simulink model "Elevator_Group_Final"  (R2020b)
settings: Solver=VariableStepAuto  StartTime=0.0  StopTime=100  RelTol=1e-3
libraries: vrlib x6
settings Model: SimulationMode=accelerator  EnablePacing=on  Creator=eric  LastModifiedBy=eric

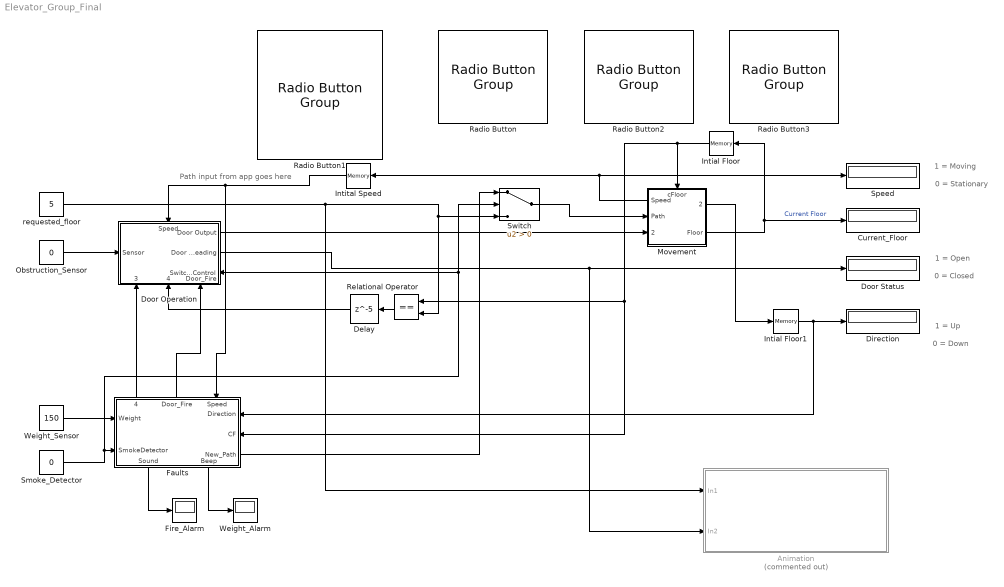
== system Elevator_Group_Final ==
  note: 0 = Closed
  note: 1 = Open
  note: 0 = Stationary
  note: 1 = Moving
  note: 0 = Down
  note: 1 = Up
  note: Path input from app goes here
  Animation : Subsystem  Commented=on
  Current_Floor : Display
  Delay : Delay  DelayLength=5  DelayLengthUpperLimit=1  InitialCondition=5
  Direction : Display
  Door Operation : Subsystem
      settings: PortSchema="{\"entries\":[{\"content\":{\"sides\":[{\"content\":{\"connectorIds\":[\"In1\"]},\"type\":\"ConnectorPlacement.EquallySpacedRectSide\",\"uuid\":\"30977b0a-2af7-4c61-bebb-4ec80410b903\"},{\"content\":{\"connectorIds\":[\"Out1\",\"Out2\",\"In6\"],\"side\":\"RIGHT\"},\"type\":\"ConnectorPlacement.EquallySpacedRectSide\",\"uuid\":\"323388e5-4c35-430e-8d9e-2a05895b747e\"},{\"content\":{\"connectorIds\":[\"In2\"],\"side\":\"TOP\"},\"type\":\"ConnectorPlacement.EquallySpacedRectSide\",\"uuid\":\"9d5d1b04-f04c-4d1c-b5e3-f520ce15ffef\"},{\"content\":{\"connectorIds\":[\"In3\",\"In4\",\"In5\"],\"side\":\"BOTTOM\"},\"type\":\"ConnectorPlacement.EquallySpacedRectSide\",\"uuid\":\"a2796d79-cbcd-43fd-84cb-bc57d429544b\"},{\"content\":{\"connectorIds\":[],\"side\":\"HIDDEN\"},\"type\":\"ConnectorPlacement.EquallySpacedRectSide\",\"uuid\":\"d7ca2218-6b24-4bda-a0e6-55c9b81b1772\"}]},\"type\":\"ConnectorPlacement.EquallySpacedConnector\",\"uuid\":\"8cf9c2d5-6e60-4b33-b84b-36b0ae7fd4c7\"}],\"packageUris\":[\"http://schema.mathworks.com/mf0/Connector/R2020b\"],\"version\":\"1.0\"}"
  Door Status : Display
      settings: Format=decimal (Stored Integer)
  Faults : Subsystem
      settings: PortSchema="{\"entries\":[{\"content\":{\"sides\":[{\"content\":{\"connectorIds\":[\"In1\",\"In2\"]},\"type\":\"ConnectorPlacement.EquallySpacedRectSide\",\"uuid\":\"b542c6e3-be07-4424-9acd-05bcaa8665d0\"},{\"content\":{\"connectorIds\":[\"In4\",\"In5\",\"Out1\"],\"side\":\"RIGHT\"},\"type\":\"ConnectorPlacement.EquallySpacedRectSide\",\"uuid\":\"4c454740-b190-4de2-b331-8e0c80643a87\"},{\"content\":{\"connectorIds\":[\"Out4\",\"Out5\",\"In3\"],\"side\":\"TOP\"},\"type\":\"ConnectorPlacement.EquallySpacedRectSide\",\"uuid\":\"6729b97a-e3fb-490d-b4f5-469d78231d99\"},{\"content\":{\"connectorIds\":[\"Out2\",\"Out3\"],\"side\":\"BOTTOM\"},\"type\":\"ConnectorPlacement.EquallySpacedRectSide\",\"uuid\":\"d3dc2118-b61f-4cf9-a6c5-d526f7b388be\"},{\"content\":{\"connectorIds\":[],\"side\":\"HIDDEN\"},\"type\":\"ConnectorPlacement.EquallySpacedRectSide\",\"uuid\":\"1ff5b4e2-fa65-45ee-8266-e12ec9f62a5d\"}]},\"type\":\"ConnectorPlacement.EquallySpacedConnector\",\"uuid\":\"a702394a-464a-4810-a0b3-3c736674cde3\"}],\"packageUris\":[\"http://schema.mathworks.com/mf0/Connector/R2020b\"],\"version\":\"1.0\"}"
  Fire_Alarm : Display
  Intial Floor : Memory
  Intial Floor1 : Memory  InitialCondition=1
  Intital Speed : Memory
  Movement : Stateflow chart  TreatAsAtomicUnit=on
      settings: PortSchema="{\"entries\":[{\"content\":{\"sides\":[{\"content\":{\"connectorIds\":[\"Out1\",\"In3\",\"In2\"]},\"type\":\"ConnectorPlacement.EquallySpacedRectSide\",\"uuid\":\"723fcccf-a5ea-4524-a847-31e47b2c7577\"},{\"content\":{\"connectorIds\":[\"Out2\",\"Out3\"],\"side\":\"RIGHT\"},\"type\":\"ConnectorPlacement.EquallySpacedRectSide\",\"uuid\":\"c79bb0ca-7135-417f-bf20-d4a9209b0782\"},{\"content\":{\"connectorIds\":[\"In1\"],\"side\":\"TOP\"},\"type\":\"ConnectorPlacement.EquallySpacedRectSide\",\"uuid\":\"4a8db4cf-0e92-4abd-a983-fa8b3d66675d\"},{\"content\":{\"connectorIds\":[],\"side\":\"HIDDEN\"},\"type\":\"ConnectorPlacement.EquallySpacedRectSide\",\"uuid\":\"59d7251f-75ad-48da-8ece-7fda6e08ec45\"}]},\"type\":\"ConnectorPlacement.EquallySpacedConnector\",\"uuid\":\"c629af32-1ebf-4e2d-97c9-9fb50af07127\"}],\"packageUris\":[\"http://schema.mathworks.com/mf0/Connector/R2020b\"],\"version\":\"1.0\"}"
  Obstruction_Sensor : Constant  Value=0
  Radio Button : RadioButtonGroup  SelectedLabel=No Obstruction  ButtonGroupName=Sensor
      settings: Values={{'No Obstruction', 'Obstruction'}, [0 1]}
  Radio Button1 : RadioButtonGroup  SelectedLabel=5  ButtonGroupName=Floor
      settings: Values={{'0', '1', '2', '3', '4', '5'}, [0 1 2 3 4 5]}
  Radio Button2 : RadioButtonGroup  SelectedLabel=150kg  ButtonGroupName=Weight
      settings: Values={{'0kg', '150kg', '300kg (Overweight)', '400kg (Overweight)'}, [0 150 300 400]}
  Radio Button3 : RadioButtonGroup  SelectedLabel=No Smoke  ButtonGroupName=Smoke Detector
      settings: Values={{'No Smoke', 'Smoke'}, [0 1]}
  Relational Operator : RelationalOperator  Operator===  OutDataTypeStr=boolean  RndMeth=Simplest
  Smoke_Detector : Constant  Value=0
  Speed : Display
      settings: Format=decimal (Stored Integer)
  Switch : Switch  Criteria=u2 > Threshold
  Weight_Alarm : Display
  Weight_Sensor : Constant  Value=150
  requested_floor : Constant  Value=5
  wires:
  Movement/3(Floor) -> Intial Floor/1, Current_Floor/1  "Current Floor"
  Movement/1(Speed) -> Intital Speed/1, Speed/1
  Intial Floor/1 -> Faults/5(CF), Relational Operator/1, Movement/1(cFloor)
  Intital Speed/1 -> Faults/3(Speed), Door Operation/2(Speed)
  Obstruction_Sensor/1 -> Door Operation/1(Sensor)
  Movement/2(Direction) -> Intial Floor1/1
  Relational Operator/1 -> Delay/1
  Delay/1 -> Door Operation/4(Delay Control)
  Door Operation/1(Door Output) -> Movement/2(Door_Output)
  Smoke_Detector/1 -> Faults/2(SmokeDetector), Switch/2, Door Operation/6(Switch Control)
  Switch/1 -> Movement/3(Path)
  Intial Floor1/1 -> Faults/4(Direction), Direction/1
  Weight_Sensor/1 -> Faults/1(Weight)
  Faults/1(New_Path) -> Switch/1
  Faults/4(Weight_Output) -> Door Operation/3(Weight_Output)
  Faults/5(Door_Fire) -> Door Operation/5(Door_Fire)
  Faults/3(Beep) -> Weight_Alarm/1
  Faults/2(Sound) -> Fire_Alarm/1
  requested_floor/1 -> Animation/1(In1), Switch/3, Relational Operator/2
  Door Operation/2(Door Reading) -> Animation/2(In2), Door Status/1

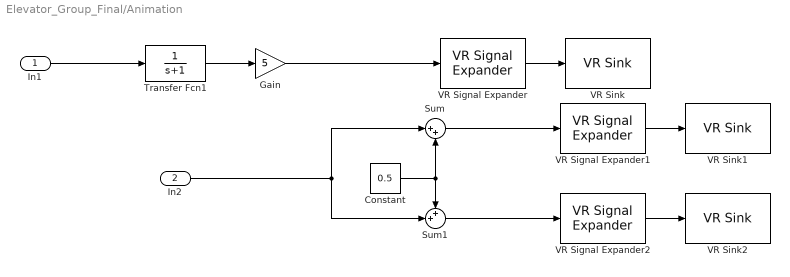
== system Elevator_Group_Final/Animation ==
  In1 : Inport
  In2 : Inport  Port=2
  Constant : Constant  Value=0.5
  Gain : Gain  Gain=5
  Sum : Sum  Inputs=|++
  Sum1 : Sum  Inputs=++|
  Transfer Fcn1 : TransferFcn  Denominator=[1 1]
  VR Signal Expander : vrlib/VR Signal Expander  outwidth=3  outidx=[2]
  VR Signal Expander1 : vrlib/VR Signal Expander  outwidth=3  outidx=[1]
  VR Signal Expander2 : vrlib/VR Signal Expander  outwidth=3  outidx=[1]
  VR Sink : vrlib/VR Sink  InstantiateOnLoad=on  SampleTime=0.01  ViewEnable=on  RemoteChange=off  RemoteView=off  FieldsWritten=box.translation.3.1.1.double  WorldFileName=elevator model.x3d  AutoView=off  VideoDimensions=[]  AllowVariableSize=off
  VR Sink1 : vrlib/VR Sink  InstantiateOnLoad=on  SampleTime=0.01  ViewEnable=on  RemoteChange=off  RemoteView=off  FieldsWritten=Door_L.translation.3.1.1.double  WorldFileName=elevator model.x3d  AutoView=off  VideoDimensions=[]  AllowVariableSize=off
  VR Sink2 : vrlib/VR Sink  InstantiateOnLoad=on  SampleTime=0.01  ViewEnable=on  RemoteChange=off  RemoteView=off  FieldsWritten=Door_R.translation.3.1.1.double  WorldFileName=elevator model.x3d  AutoView=off  VideoDimensions=[]  AllowVariableSize=off
  wires:
  In1/1 -> Transfer Fcn1/1
  Gain/1 -> VR Signal Expander/1
  VR Signal Expander1/1 -> VR Sink1/1
  Constant/1 -> Sum1/1, Sum/2
  In2/1 -> Sum/1, Sum1/2
  Sum1/1 -> VR Signal Expander2/1
  Sum/1 -> VR Signal Expander1/1
  VR Signal Expander2/1 -> VR Sink2/1
  Transfer Fcn1/1 -> Gain/1
  VR Signal Expander/1 -> VR Sink/1

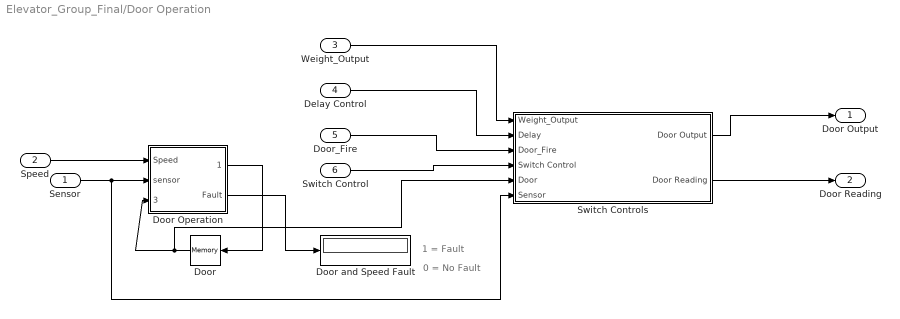
== system Elevator_Group_Final/Door Operation ==
  note: 0 = No Fault
  note: 1 = Fault
  Sensor : Inport
  Speed : Inport  Port=2  OutMin=0  OutMax=2  OutDataTypeStr=double
  Weight_Output : Inport  Port=3
  Delay Control : Inport  Port=4
  Door_Fire : Inport  Port=5
  Switch Control : Inport  Port=6
  Door : Memory  InitialCondition=1  InheritSampleTime=on  LinearizeMemory=on
  Door Operation : Stateflow chart  TreatAsAtomicUnit=on
      settings: PortSchema="{\"entries\":[{\"content\":{\"sides\":[{\"content\":{\"connectorIds\":[\"In2\",\"In1\",\"In3\"]},\"type\":\"ConnectorPlacement.EquallySpacedRectSide\",\"uuid\":\"31e92d3c-0266-4042-9cc0-73e2fa5475a5\"},{\"content\":{\"connectorIds\":[\"Out1\",\"Out2\"],\"side\":\"RIGHT\"},\"type\":\"ConnectorPlacement.EquallySpacedRectSide\",\"uuid\":\"0ce7aa6e-b975-49b3-b309-422d5642910d\"},{\"content\":{\"connectorIds\":[],\"side\":\"TOP\"},\"type\":\"ConnectorPlacement.EquallySpacedRectSide\",\"uuid\":\"d77baac7-bcfc-4c97-8f5f-a05c60ec2b96\"},{\"content\":{\"connectorIds\":[],\"side\":\"HIDDEN\"},\"type\":\"ConnectorPlacement.EquallySpacedRectSide\",\"uuid\":\"7d61dd79-ac27-4838-8e0e-1c25083bca29\"}]},\"type\":\"ConnectorPlacement.EquallySpacedConnector\",\"uuid\":\"ed20ea32-9081-4fe8-8264-861068f1e86e\"}],\"packageUris\":[\"http://schema.mathworks.com/mf0/Connector/R2020b\"],\"version\":\"1.0\"}"
  Door and Speed Fault : Display
  Switch Controls : Subsystem
  Door Output : Outport
  Door Reading : Outport  Port=2
  wires:
  Speed/1 -> Door Operation/2(Speed)
  Sensor/1 -> Switch Controls/6(Sensor), Door Operation/1(sensor)
  Door/1 -> Switch Controls/5(Door), Door Operation/3(Door_initial)
  Door Operation/2(Fault) -> Door and Speed Fault/1
  Door Operation/1(Door_output) -> Door/1
  Door_Fire/1 -> Switch Controls/3(Door_Fire)
  Switch Control/1 -> Switch Controls/4(Switch Control)
  Delay Control/1 -> Switch Controls/2(Delay)
  Weight_Output/1 -> Switch Controls/1(Weight_Output)
  Switch Controls/1(Door Output) -> Door Output/1
  Switch Controls/2(Door Reading) -> Door Reading/1

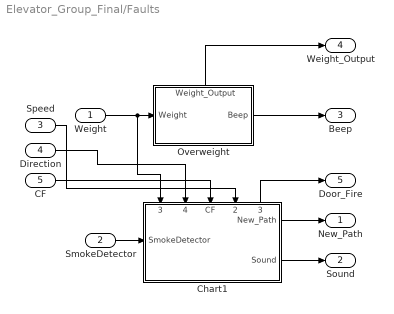
== system Elevator_Group_Final/Faults ==
  Weight : Inport
  SmokeDetector : Inport  Port=2
  Speed : Inport  Port=3
  Direction : Inport  Port=4
  CF : Inport  Port=5
  Chart1 : Stateflow chart  TreatAsAtomicUnit=on
      settings: PortSchema="{\"entries\":[{\"content\":{\"sides\":[{\"content\":{\"connectorIds\":[\"In1\"]},\"type\":\"ConnectorPlacement.EquallySpacedRectSide\",\"uuid\":\"4338b933-4c90-4296-ae2f-b7ec197f71ee\"},{\"content\":{\"connectorIds\":[\"Out1\",\"Out2\"],\"side\":\"RIGHT\"},\"type\":\"ConnectorPlacement.EquallySpacedRectSide\",\"uuid\":\"ab225833-92e6-40a0-941c-7bd795c841af\"},{\"content\":{\"connectorIds\":[\"In3\",\"In4\",\"In5\",\"In2\",\"Out3\"],\"side\":\"TOP\"},\"type\":\"ConnectorPlacement.EquallySpacedRectSide\",\"uuid\":\"850bf22d-2eb0-4aac-8910-ff5759bdc595\"},{\"content\":{\"connectorIds\":[],\"side\":\"HIDDEN\"},\"type\":\"ConnectorPlacement.EquallySpacedRectSide\",\"uuid\":\"2713262d-6e79-4417-8ed8-ffa624643aaa\"}]},\"type\":\"ConnectorPlacement.EquallySpacedConnector\",\"uuid\":\"85fffa3c-755d-471d-bfdb-cb1164fb2fdc\"}],\"packageUris\":[\"http://schema.mathworks.com/mf0/Connector/R2020b\"],\"version\":\"1.0\"}"
  Overweight : Stateflow chart  TreatAsAtomicUnit=on
      settings: PortSchema="{\"entries\":[{\"content\":{\"sides\":[{\"content\":{\"connectorIds\":[\"In1\"]},\"type\":\"ConnectorPlacement.EquallySpacedRectSide\",\"uuid\":\"26b51c16-ea5f-4cd9-8858-b0cd52271dc0\"},{\"content\":{\"connectorIds\":[\"Out1\"],\"side\":\"RIGHT\"},\"type\":\"ConnectorPlacement.EquallySpacedRectSide\",\"uuid\":\"53489c37-c06b-4fea-858b-14f398593ef8\"},{\"content\":{\"connectorIds\":[\"Out2\"],\"side\":\"TOP\"},\"type\":\"ConnectorPlacement.EquallySpacedRectSide\",\"uuid\":\"af0547f4-2efe-4cfd-957f-913b3db1f9eb\"},{\"content\":{\"connectorIds\":[],\"side\":\"HIDDEN\"},\"type\":\"ConnectorPlacement.EquallySpacedRectSide\",\"uuid\":\"b962f037-ab24-43a6-9e25-c96a4a0224cc\"}]},\"type\":\"ConnectorPlacement.EquallySpacedConnector\",\"uuid\":\"d04235de-47c1-4895-9e87-a3d9e0b489b1\"}],\"packageUris\":[\"http://schema.mathworks.com/mf0/Connector/R2020b\"],\"version\":\"1.0\"}"
  New_Path : Outport
  Sound : Outport  Port=2
  Beep : Outport  Port=3
  Weight_Output : Outport  Port=4
  Door_Fire : Outport  Port=5
  wires:
  Overweight/1(Beep) -> Beep/1
  Chart1/2(Sound) -> Sound/1
  Overweight/2(Weight_Output) -> Weight_Output/1
  Chart1/3(Door_Fire) -> Door_Fire/1
  Chart1/1(New_Path) -> New_Path/1
  Speed/1 -> Chart1/2(Speed)
  Direction/1 -> Chart1/4(Direction)
  SmokeDetector/1 -> Chart1/1(SmokeDetector)
  CF/1 -> Chart1/5(CF)
  Weight/1 -> Chart1/3(Weight), Overweight/1(Weight)

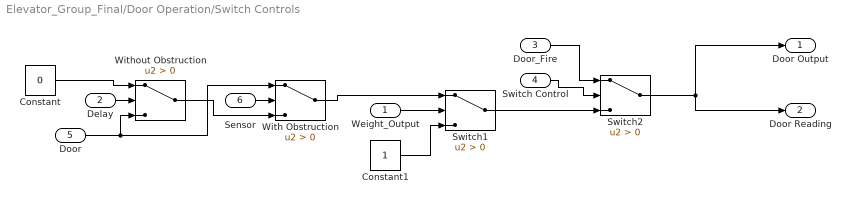
== system Elevator_Group_Final/Door Operation/Switch Controls ==
  Weight_Output : Inport
  Delay : Inport  Port=2
  Door_Fire : Inport  Port=3
  Switch Control : Inport  Port=4
  Door : Inport  Port=5
  Sensor : Inport  Port=6
  Constant : Constant  Value=0
  Constant1 : Constant
  Switch1 : Switch  Criteria=u2 > Threshold
  Switch2 : Switch  Criteria=u2 > Threshold
  With Obstruction : Switch  Criteria=u2 > Threshold
  Without Obstruction : Switch  Criteria=u2 > Threshold
  Door Output : Outport
  Door Reading : Outport  Port=2
  wires:
  Weight_Output/1 -> Switch1/2
  Switch1/1 -> Switch2/3
  Switch2/1 -> Door Reading/1, Door Output/1
  Door_Fire/1 -> Switch2/1
  Switch Control/1 -> Switch2/2
  Constant1/1 -> Switch1/3
  Delay/1 -> Without Obstruction/2
  Door/1 -> With Obstruction/1, Without Obstruction/3
  Constant/1 -> Without Obstruction/1
  Sensor/1 -> With Obstruction/2
  With Obstruction/1 -> Switch1/1
  Without Obstruction/1 -> With Obstruction/3

== stateflow chart Elevator_Group_Final/Faults/Overweight ==
  state Stay
    entry:
    Weight_Output = 0
  state Move
    entry:
    Weight_Output = 1
  (default) -> (junction 7) : {WeightLimit = 300}
  Move -> (junction 7)
  (junction 7) -> (junction 9) [order 1] : [Weight >= WeightLimit]
  Stay -> (junction 7) : [Weight<= WeightLimit]
  (junction 7) -> Move [order 2] : {Beep = 0;}
  (junction 9) -> Stay : {Beep = 1;}
  data: Beep output; Weight input; WeightLimit local; Weight_Output output

== stateflow chart Elevator_Group_Final/Door Operation/Door Operation ==
  state Idle
    en:
    Speed;
    sensor;
    Door =Door_initial;
    Door_output=Door;
    Fault = 0;
  state Arrving
    exit:
    Door= 1;
  state Fault [commented out]
    en:
    Door=0;
    Speed=0;
    Fault=1;
  state Door_Output
    en:
    after(0.5,sec);
  state Obstacle_detection
    en:
    sensor;
    after(2,sec)
  state Leaving
    exit:
    Door= 0;
  Door_Output -> Idle : [after(0.5,sec)]
  (default) -> Idle
  Idle -> Arrving [order 1] : [Door==0 & Speed==0] %end of path
  Idle -> Fault [commented out] : [Door==1& Speed > 0]
  Arrving -> Door_Output : {Door_output=1}
  Fault -> Idle [commented out] : [Door==0 & Speed==0]
  Leaving -> Door_Output : {Door_output=0}
  Idle -> Obstacle_detection [order 2] : [Door==1 & Speed==0]%start of path
  Obstacle_detection -> Leaving [order 2] : [sensor==0]
  Obstacle_detection -> Obstacle_detection [order 1] : [sensor==1]{Door_output=1}
  data: sensor input; Door_output output; Speed input; Door local; Door_initial input; Fault output

== stateflow chart Elevator_Group_Final/Movement ==
  state Idle
    en:
    Action=Path;
    Floor = cFloor;
  state Up
    en:
    Speed = 1;
    Direction = 1;
    Floor = Floor +1;
    during:
    motor=1;
    after(3,sec)
    motor= 0
  state Door_Trigger
    during:
    after(2.5,sec)
  state Down
    en:
    Speed = 1;
    Direction = 0;
    Floor = Floor -1;
    during:
    motor=1;
    after(3,sec)
    motor= 0
  Idle -> Door_Trigger [order 2] : [Action==Floor&Door_Output==1]
  Door_Trigger -> Idle [order 2] : [Door_Output == 0]
  (default) -> Idle
  Idle -> Up [order 3] : [Action>Floor & Door_Output==0]
  Door_Trigger -> Door_Trigger [order 1] : [Door_Output==1]
  Up -> Door_Trigger [order 2] : [Action==Floor]{Speed=0}
  Idle -> Idle [order 1] : [Door_Output==1]
  Idle -> Down [order 4] : [Action<Floor & Door_Output==0]
  Down -> Door_Trigger [order 2] : [Action==Floor]{Speed=0}
  Up -> Up [order 1] : [Floor~=Action]
  Down -> Down [order 1] : [Floor~=Action]
  data: cFloor input; Speed output; Door_Output input; Path input; Action local; motor local; Direction output; Floor output

== stateflow chart Elevator_Group_Final/Faults/Chart1 ==
  state Check
    en:
    Alarm=0;
  state FireAlarm
    state StopElevator
      state GoingDown
        entry:
        New_Path = CF - 1
      state GoingUp
        entry:
        New_Path = CF + 1
      (default) -> (junction 42)
      (junction 42) -> GoingDown [order 2]
      (junction 42) -> GoingUp [order 1] : [Direction == 1]
    state OpenDoor
      entry:
      Door_Fire = 1
      Alarm = 1
    state ShutDown
      entry:
      Door_Fire = 0
      ShutDown = 1
    (default) -> (junction 18) : {Sound = 1}
    (junction 18) -> StopElevator [order 1] : [Speed == 1]
    (junction 18) -> (junction 29) [order 2] : {New_Path = CF}
    (junction 29) -> OpenDoor [order 1] : [Weight > 0]
    StopElevator -> (junction 29) : [New_Path == CF]
    (junction 29) -> ShutDown [order 2]
    OpenDoor -> ShutDown : after (10,sec) [Weight == 0]
  (default) -> Check
  Check -> Check [order 2]
  Check -> FireAlarm [order 1] : [SmokeDetector == 1]
  data: SmokeDetector input; New_Path output; Speed input; Weight input; Direction input; CF input; ShutDown local; Sound output; Alarm local; Door_Fire output
